simulink model "RequirementsTable"  (R2023a)
settings: Solver=FixedStepDiscrete  StartTime=0.0  StopTime=10.0  RelTol=1e-3
settings Model: DVExtractedSubsystem=Requirements Table  DVDesignModelName=MioProgetto  Creator=bened  LastModifiedBy=bened
settings SolverCC: MaxZcPerStep=1
settings DebuggingCC: UnconnectedInputMsg=warning  UnconnectedOutputMsg=warning  UnconnectedLineMsg=warning  FrameProcessingCompatibilityMsg=none
settings ModelReferenceCC: EnableRefExpFcnMdlSchedulingChecks=on
settings RTWCC: TLCOptions=-aAlwaysIncludeCustomSrc=1  DLArmComputeVersion=19.05

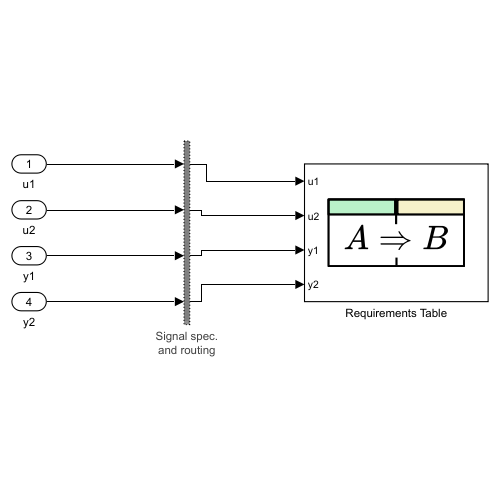
[thumbnail: Simulink's stored preview of the top-level diagram]
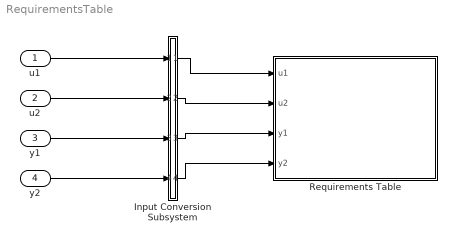
== system RequirementsTable ==
  u1 : Inport  OutDataTypeStr=double  PortDimensions=[1]  SampleTime=[-1, 0]  Interpolate=off
  u2 : Inport  Port=2  OutDataTypeStr=double  PortDimensions=[1]  SampleTime=[-1, 0]  Interpolate=off
  y1 : Inport  Port=3  OutDataTypeStr=double  PortDimensions=[1]  SampleTime=[-1, 0]  Interpolate=off
  y2 : Inport  Port=4  OutDataTypeStr=double  PortDimensions=[1]  SampleTime=[-1, 0]  Interpolate=off
  Input Conversion Subsystem : Subsystem  Tag=__SLT_ICS__  Description=|
      | Signal spec.
      | and routing
      settings: AttributesFormatString=%<Description>
  Requirements Table : Requirements Table  TreatAsAtomicUnit=on
  wires:
  u1/1 -> Input Conversion Subsystem/1(Inport_1)
  u2/1 -> Input Conversion Subsystem/2(Inport_2)
  y1/1 -> Input Conversion Subsystem/3(Inport_3)
  y2/1 -> Input Conversion Subsystem/4(Inport_4)
  Input Conversion Subsystem/1(Outport_1) -> Requirements Table/1(u1)
  Input Conversion Subsystem/2(Outport_2) -> Requirements Table/2(u2)
  Input Conversion Subsystem/3(Outport_3) -> Requirements Table/3(y1)
  Input Conversion Subsystem/4(Outport_4) -> Requirements Table/4(y2)

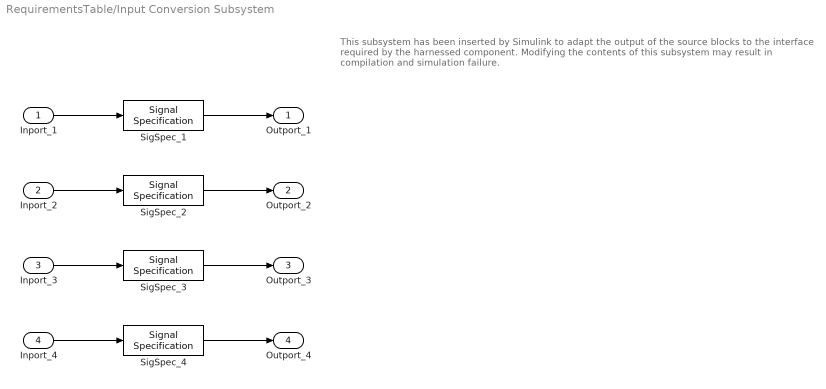
== system RequirementsTable/Input Conversion Subsystem ==
  note: This subsystem has been inserted by Simulink to adapt the output of the source blocks to the interface required by the harnessed component.
      |  Modifying the contents of this subsystem may result in compilation and simulation failure.
  Inport_1 : Inport
  Inport_2 : Inport  Port=2
  Inport_3 : Inport  Port=3
  Inport_4 : Inport  Port=4
  SigSpec_{1..4} (4 alike) : SignalSpecification  OutDataTypeStr=double  Dimensions=[1]  SampleTime=[-1, 0]
  Outport_1 : Outport
  Outport_2 : Outport  Port=2
  Outport_3 : Outport  Port=3
  Outport_4 : Outport  Port=4
  wires:
  SigSpec_1/1 -> Outport_1/1
  Inport_1/1 -> SigSpec_1/1
  SigSpec_2/1 -> Outport_2/1
  Inport_2/1 -> SigSpec_2/1
  SigSpec_3/1 -> Outport_3/1
  Inport_3/1 -> SigSpec_3/1
  SigSpec_4/1 -> Outport_4/1
  Inport_4/1 -> SigSpec_4/1

== stateflow chart RequirementsTable/Requirements Table ==
  (default) -> (junction 1073742737)
  (junction 1073742737) -> (junction 1073742738) : {
      | % SF_REQ_REV_07
      | }
  (junction 1073742738) -> (junction 1073742740) : {
      | % HEADER_ASSIGNMENTS
      |
      | }
  (junction 1073742740) -> (junction 1073742742) : {
      | % START_A_4
      | }
  (junction 1073742742) -> (junction 1073742744) : {
      | }
  (junction 1073742744) -> (junction 1073742746)
  (junction 1073742746) -> (junction 1073742748) : {
      | }
  (junction 1073742748) -> (junction 1073742750) : {
      | % END_A_4
      | }
  (junction 1073742750) -> (junction 1073742752) : {
      | % START_R_7
      | }
  (junction 1073742752) -> (junction 1073742754) : {
      | }
  (junction 1073742754) -> (junction 1073742756)
  (junction 1073742756) -> (junction 1073742758) [order 1] : [(u1==prev(u1)+1)]
  (junction 1073742756) -> (junction 1073742764) [order 2]
  (junction 1073742758) -> (junction 1073742760) : {
      | reqtable_postcondition((y1 == y1+2), 'R:1');
      |
      |
      | }
  (junction 1073742760) -> (junction 1073742762) : {
      | }
  (junction 1073742762) -> (junction 1073742764)
  (junction 1073742764) -> (junction 1073742766)
  (junction 1073742766) -> (junction 1073742768) : {
      | % END_R_7
      | }
  (junction 1073742768) -> (junction 1073742770) : {
      | % START_R_1
      | }
  (junction 1073742770) -> (junction 1073742772) : {
      | }
  (junction 1073742772) -> (junction 1073742774)
  (junction 1073742774) -> (junction 1073742776) [order 1] : [(u2 > 2)]
  (junction 1073742774) -> (junction 1073742782) [order 2]
  (junction 1073742776) -> (junction 1073742778) : {
      |
      |
      | }
  (junction 1073742778) -> (junction 1073742780) : {
      | }
  (junction 1073742780) -> (junction 1073742782)
  (junction 1073742782) -> (junction 1073742784)
  (junction 1073742784) -> (junction 1073742786) : {
      | % END_R_1
      | }
  data: u1 input; u2 input; y1 input; y2 input
